simulink model "Quadrotor_Simulation"  (R2016b)
settings: Solver=VariableStepAuto  StartTime=0.0  StopTime=15  FixedStep=0.005  MaxStep=0.005  RelTol=1e-1
settings Model: Creator=Administrator  LastModifiedBy=Administrator

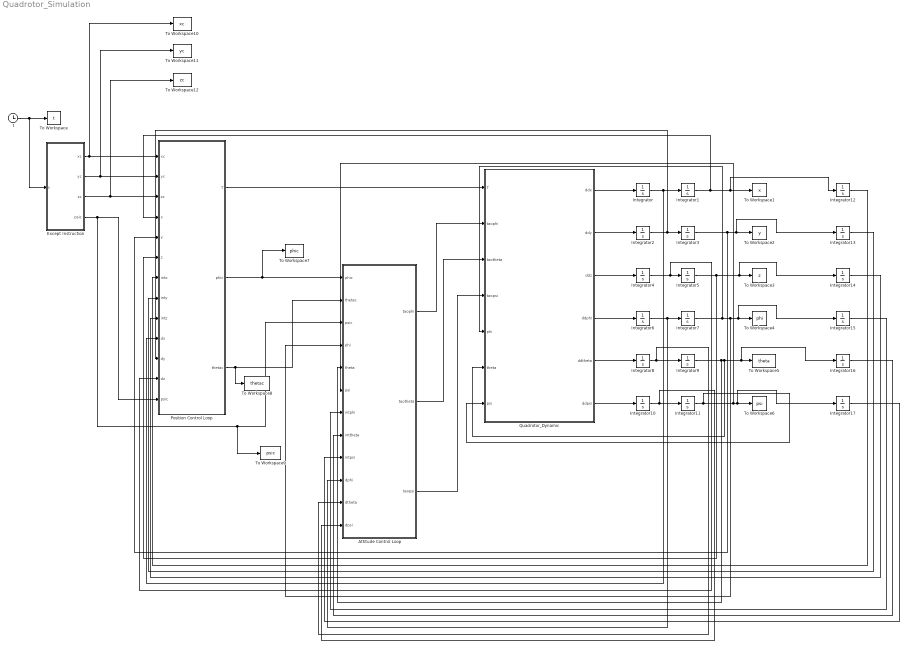
== system Quadrotor_Simulation ==
  Attitude Control Loop : Subsystem
  Except Instruction : MATLAB Function  TreatAsAtomicUnit=on
  Integrator : Integrator  InitialCondition=0.1
  Integrator{1,3,5..17} (15 alike) : Integrator
  Integrator2 : Integrator  InitialCondition=0.1
  Integrator4 : Integrator  InitialCondition=0.1
  Position Control Loop : Subsystem
  Quadrotor_Dynamic : MATLAB Function  TreatAsAtomicUnit=on
  To Workspace : ToWorkspace  VariableName=t  SampleTime=-1
  To Workspace1 : ToWorkspace  VariableName=x  SampleTime=-1
  To Workspace10 : ToWorkspace  VariableName=xc  SampleTime=-1
  To Workspace11 : ToWorkspace  VariableName=yc  SampleTime=-1
  To Workspace12 : ToWorkspace  VariableName=zc  SampleTime=-1
  To Workspace2 : ToWorkspace  VariableName=y  SampleTime=-1
  To Workspace3 : ToWorkspace  VariableName=z  SampleTime=-1
  To Workspace4 : ToWorkspace  VariableName=phi  SampleTime=-1
  To Workspace5 : ToWorkspace  VariableName=theta  SampleTime=-1
  To Workspace6 : ToWorkspace  VariableName=psi  SampleTime=-1
  To Workspace7 : ToWorkspace  VariableName=phic  SampleTime=-1
  To Workspace8 : ToWorkspace  VariableName=thetac  SampleTime=-1
  To Workspace9 : ToWorkspace  VariableName=psic  SampleTime=-1
  t : Clock
  wires:
  t/1 -> Except Instruction/1(t), To Workspace/1
  Except Instruction/1(xc) -> To Workspace10/1, Position Control Loop/1(xc)
  Except Instruction/2(yc) -> To Workspace11/1, Position Control Loop/2(yc)
  Except Instruction/3(zc) -> To Workspace12/1, Position Control Loop/3(zc)
  Except Instruction/4(psic) -> Attitude Control Loop/3(psic), To Workspace9/1, Position Control Loop/13(psic)
  Position Control Loop/2(phic) -> To Workspace7/1, Attitude Control Loop/1(phic)
  Position Control Loop/3(thetac) -> To Workspace8/1, Attitude Control Loop/2(thetac)
  Quadrotor_Dynamic/1(ddx) -> Integrator/1
  Integrator/1 -> Position Control Loop/10(dx), Integrator1/1
  Quadrotor_Dynamic/2(ddy) -> Integrator2/1
  Integrator2/1 -> Integrator3/1, Position Control Loop/11(dy)
  Quadrotor_Dynamic/3(ddz) -> Integrator4/1
  Integrator4/1 -> Position Control Loop/12(dz), Integrator5/1
  Quadrotor_Dynamic/4(ddphi) -> Integrator6/1
  Integrator6/1 -> Attitude Control Loop/10(dphi), Integrator7/1
  Quadrotor_Dynamic/5(ddtheta) -> Integrator8/1
  Integrator8/1 -> Attitude Control Loop/11(dtheta), Integrator9/1
  Quadrotor_Dynamic/6(ddpsi) -> Integrator10/1
  Integrator10/1 -> Attitude Control Loop/12(dpsi), Integrator11/1
  Integrator9/1 -> Attitude Control Loop/5(theta), Quadrotor_Dynamic/6(theta), Integrator16/1, To Workspace5/1
  Integrator11/1 -> Quadrotor_Dynamic/7(psi), Integrator17/1, To Workspace6/1, Attitude Control Loop/6(psi)
  Integrator7/1 -> Quadrotor_Dynamic/5(phi), Attitude Control Loop/4(phi), Integrator15/1, To Workspace4/1
  Integrator5/1 -> Position Control Loop/6(z), Integrator14/1, To Workspace3/1
  Integrator3/1 -> Position Control Loop/5(y), Integrator13/1, To Workspace2/1
  Integrator1/1 -> Position Control Loop/4(x), Integrator12/1, To Workspace1/1
  Position Control Loop/1(T) -> Quadrotor_Dynamic/1(T)
  Attitude Control Loop/1(taophi) -> Quadrotor_Dynamic/2(taophi)
  Attitude Control Loop/2(taotheta) -> Quadrotor_Dynamic/3(taotheta)
  Attitude Control Loop/3(taopsi) -> Quadrotor_Dynamic/4(taopsi)
  Integrator12/1 -> Position Control Loop/7(intx)
  Integrator13/1 -> Position Control Loop/8(inty)
  Integrator14/1 -> Position Control Loop/9(intz)
  Integrator15/1 -> Attitude Control Loop/7(intphi)
  Integrator16/1 -> Attitude Control Loop/8(inttheta)
  Integrator17/1 -> Attitude Control Loop/9(intpsi)

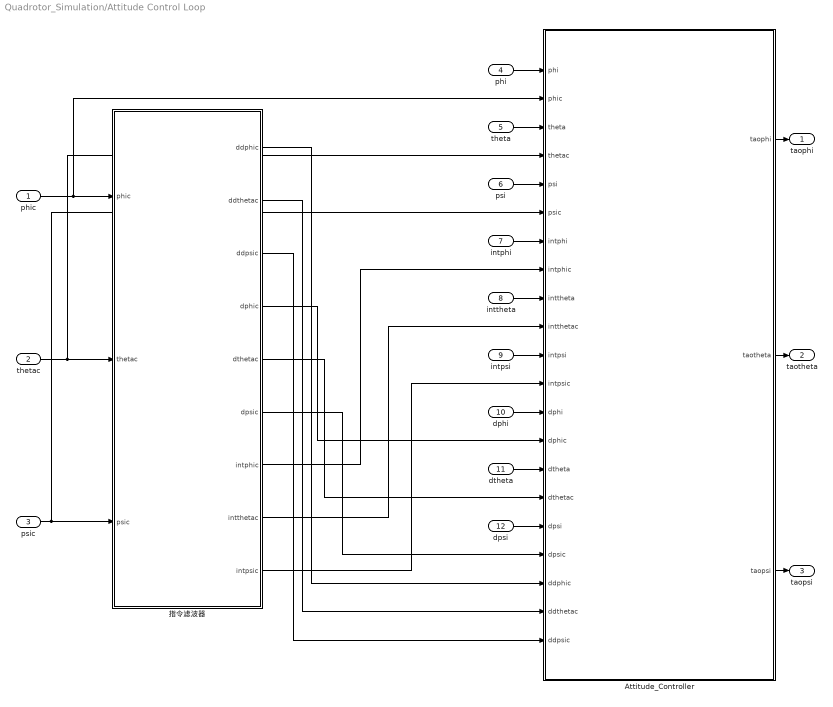
== system Quadrotor_Simulation/Attitude Control Loop ==
  phic : Inport
  thetac : Inport  Port=2
  psic : Inport  Port=3
  phi : Inport  Port=4
  theta : Inport  Port=5
  psi : Inport  Port=6
  intphi : Inport  Port=7
  inttheta : Inport  Port=8
  intpsi : Inport  Port=9
  dphi : Inport  Port=10
  dtheta : Inport  Port=11
  dpsi : Inport  Port=12
  Attitude_Controller : MATLAB Function  TreatAsAtomicUnit=on
  指令滤波器 : Subsystem
  taophi : Outport
  taotheta : Outport  Port=2
  taopsi : Outport  Port=3
  wires:
  指令滤波器/9(intpsic) -> Attitude_Controller/12(intpsic)
  指令滤波器/4(dphic) -> Attitude_Controller/14(dphic)
  dtheta/1 -> Attitude_Controller/15(dtheta)
  theta/1 -> Attitude_Controller/3(theta)
  dphi/1 -> Attitude_Controller/13(dphi)
  thetac/1 -> Attitude_Controller/4(thetac), 指令滤波器/2(thetac)
  inttheta/1 -> Attitude_Controller/9(inttheta)
  指令滤波器/7(intphic) -> Attitude_Controller/8(intphic)
  指令滤波器/5(dthetac) -> Attitude_Controller/16(dthetac)
  dpsi/1 -> Attitude_Controller/17(dpsi)
  指令滤波器/6(dpsic) -> Attitude_Controller/18(dpsic)
  指令滤波器/1(ddphic) -> Attitude_Controller/19(ddphic)
  phic/1 -> Attitude_Controller/2(phic), 指令滤波器/1(phic)
  phi/1 -> Attitude_Controller/1(phi)
  指令滤波器/8(intthetac) -> Attitude_Controller/10(intthetac)
  psi/1 -> Attitude_Controller/5(psi)
  psic/1 -> Attitude_Controller/6(psic), 指令滤波器/3(psic)
  intpsi/1 -> Attitude_Controller/11(intpsi)
  指令滤波器/3(ddpsic) -> Attitude_Controller/21(ddpsic)
  Attitude_Controller/2(taotheta) -> taotheta/1
  Attitude_Controller/3(taopsi) -> taopsi/1
  指令滤波器/2(ddthetac) -> Attitude_Controller/20(ddthetac)
  Attitude_Controller/1(taophi) -> taophi/1
  intphi/1 -> Attitude_Controller/7(intphi)

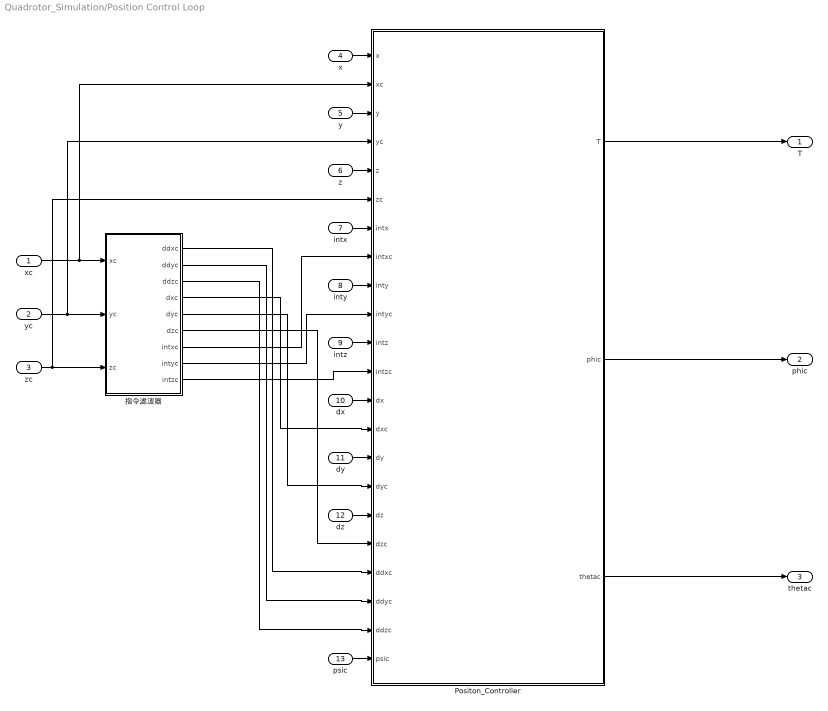
== system Quadrotor_Simulation/Position Control Loop ==
  xc : Inport
  yc : Inport  Port=2
  zc : Inport  Port=3
  x : Inport  Port=4
  y : Inport  Port=5
  z : Inport  Port=6
  intx : Inport  Port=7
  inty : Inport  Port=8
  intz : Inport  Port=9
  dx : Inport  Port=10
  dy : Inport  Port=11
  dz : Inport  Port=12
  psic : Inport  Port=13
  Positon_Controller : MATLAB Function  TreatAsAtomicUnit=on
  指令滤波器 : Subsystem
  T : Outport
  phic : Outport  Port=2
  thetac : Outport  Port=3
  wires:
  zc/1 -> Positon_Controller/6(zc), 指令滤波器/3(zc)
  yc/1 -> Positon_Controller/4(yc), 指令滤波器/2(yc)
  xc/1 -> Positon_Controller/2(xc), 指令滤波器/1(xc)
  指令滤波器/6(dzc) -> Positon_Controller/18(dzc)
  指令滤波器/8(intyc) -> Positon_Controller/10(intyc)
  指令滤波器/3(ddzc) -> Positon_Controller/21(ddzc)
  指令滤波器/7(intxc) -> Positon_Controller/8(intxc)
  指令滤波器/4(dxc) -> Positon_Controller/14(dxc)
  指令滤波器/1(ddxc) -> Positon_Controller/19(ddxc)
  指令滤波器/9(intzc) -> Positon_Controller/12(intzc)
  指令滤波器/2(ddyc) -> Positon_Controller/20(ddyc)
  指令滤波器/5(dyc) -> Positon_Controller/16(dyc)
  Positon_Controller/2(phic) -> phic/1
  Positon_Controller/3(thetac) -> thetac/1
  Positon_Controller/1(T) -> T/1
  x/1 -> Positon_Controller/1(x)
  y/1 -> Positon_Controller/3(y)
  z/1 -> Positon_Controller/5(z)
  intx/1 -> Positon_Controller/7(intx)
  inty/1 -> Positon_Controller/9(inty)
  intz/1 -> Positon_Controller/11(intz)
  dx/1 -> Positon_Controller/13(dx)
  dy/1 -> Positon_Controller/15(dy)
  dz/1 -> Positon_Controller/17(dz)
  psic/1 -> Positon_Controller/22(psic)

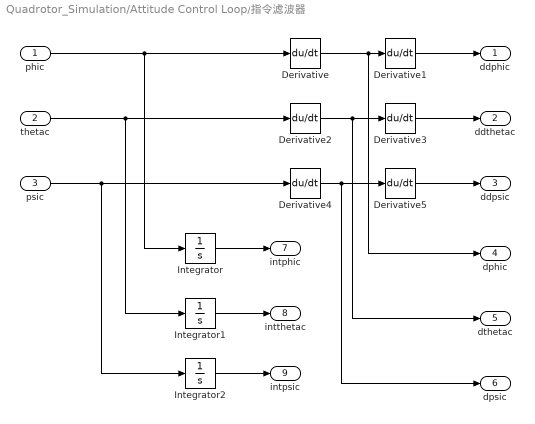
== system Quadrotor_Simulation/Attitude Control Loop/指令滤波器 ==
  phic : Inport
  thetac : Inport  Port=2
  psic : Inport  Port=3
  Derivative{,1..5} (6 alike) : Derivative
  Integrator : Integrator
  Integrator1 : Integrator
  Integrator2 : Integrator
  ddphic : Outport
  ddthetac : Outport  Port=2
  ddpsic : Outport  Port=3
  dphic : Outport  Port=4
  dthetac : Outport  Port=5
  dpsic : Outport  Port=6
  intphic : Outport  Port=7
  intthetac : Outport  Port=8
  intpsic : Outport  Port=9
  wires:
  Derivative3/1 -> ddthetac/1
  Derivative5/1 -> ddpsic/1
  Derivative1/1 -> ddphic/1
  thetac/1 -> Integrator1/1, Derivative2/1
  psic/1 -> Integrator2/1, Derivative4/1
  Derivative2/1 -> dthetac/1, Derivative3/1
  Derivative4/1 -> dpsic/1, Derivative5/1
  Derivative/1 -> dphic/1, Derivative1/1
  Integrator/1 -> intphic/1
  Integrator1/1 -> intthetac/1
  Integrator2/1 -> intpsic/1
  phic/1 -> Integrator/1, Derivative/1

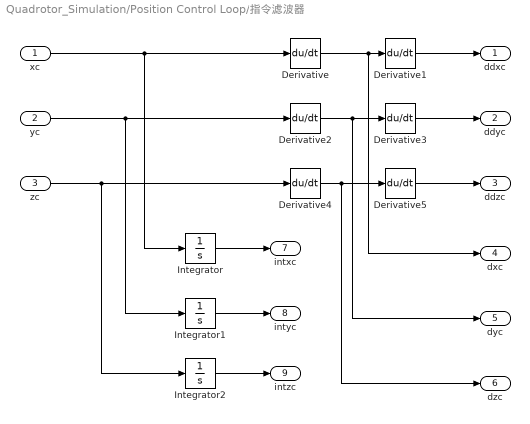
== system Quadrotor_Simulation/Position Control Loop/指令滤波器 ==
  xc : Inport
  yc : Inport  Port=2
  zc : Inport  Port=3
  Derivative{,1..5} (6 alike) : Derivative
  Integrator : Integrator
  Integrator1 : Integrator
  Integrator2 : Integrator
  ddxc : Outport
  ddyc : Outport  Port=2
  ddzc : Outport  Port=3
  dxc : Outport  Port=4
  dyc : Outport  Port=5
  dzc : Outport  Port=6
  intxc : Outport  Port=7
  intyc : Outport  Port=8
  intzc : Outport  Port=9
  wires:
  Derivative3/1 -> ddyc/1
  Derivative5/1 -> ddzc/1
  Derivative1/1 -> ddxc/1
  yc/1 -> Integrator1/1, Derivative2/1
  zc/1 -> Integrator2/1, Derivative4/1
  Derivative2/1 -> dyc/1, Derivative3/1
  Derivative4/1 -> dzc/1, Derivative5/1
  Derivative/1 -> dxc/1, Derivative1/1
  Integrator/1 -> intxc/1
  Integrator1/1 -> intyc/1
  Integrator2/1 -> intzc/1
  xc/1 -> Integrator/1, Derivative/1

== matlab function Quadrotor_Simulation/Position Control Loop/Positon_Controller ==
  data: x input; T output; xc input; y input; yc input; z input; zc input; intx input; intxc input; inty input; intyc input; intz input; intzc input; dx input; dxc input; dy input; dyc input; dz input; dzc input; ddxc input; ddyc input; ddzc input; phic output; thetac output; psic input
function [T,phic,thetac] = fcn(x,xc,y,yc,z,zc,intx,intxc,inty,intyc,intz,intzc,dx,dxc,dy,dyc,dz,dzc,ddxc,ddyc,ddzc,psic)

m = 1;
g = 9.81;

kp = 3;
ki = 0.13;
kd = 1.1;

kpx =  kp; kpy =  kp; kpz =  kp;
kix = ki; kiy = ki; kiz = ki; 
kdx = kd; kdy = kd; kdz = kd;

ex= xc - x;
ey = yc - y;
ez = zc - z;

intex = intxc - intx;
intey = intyc - inty;
intez = intzc - intz;

dex = dxc - dx;
dey = dyc - dy;
dez = dzc - dz;

%%
ddxc = 0; ddyc = 0; ddzc = 0;
%%

Ux = kpx * ex + kix * intex + kdx * dex + ddxc;
Uy = kpy * ey + kiy * intey + kdy * dey + ddyc;
Uz = kpz * ez + kiz * intez + kdz * dez + ddzc;

T = m * sqrt(Ux * Ux + Uy * Uy + (Uz + g) * (Uz + g));

temp1 = m * (Ux * sin(psic) - Uy * cos(psic)) / T;
% if temp1 > 1
%     temp1 = 1;
% elseif temp1 < -1
%     temp1 = -1;
% end
phic = asin(temp1);
% if phic > 20 * pi / 180;
%     phic = 20 * pi / 180;
% elseif phic < -20 * pi / 180
%     phic = -20 * pi / 180;
% end

temp2 = (m * Ux - T * sin(psic) * sin(phic)) / (T * cos(psic) * cos(phic));
% if temp2 > 1
%     temp2 = 1;
% elseif temp2 < -1
%     temp2 = -1;
% end
thetac = asin(temp2);
% if thetac > 20 * pi / 180
%     thetac = 20 * pi / 180;
% elseif thetac < -20 * pi / 180
%     thetac = -20 * pi / 180;
% end

== matlab function Quadrotor_Simulation/Except Instruction ==
  data: xc output; t input; yc output; zc output; psic output
function [xc,yc,zc,psic] = fcn(t)

xc = 5 * sin(t);
yc = 0.5 * sin(0.5 * t);
zc = 3;

psic = 0;

== matlab function Quadrotor_Simulation/Attitude Control Loop/Attitude_Controller ==
  data: phi input; taophi output; phic input; theta input; thetac input; psi input; psic input; intphi input; intphic input; inttheta input; intthetac input; intpsi input; intpsic input; dphi input; dphic input; dtheta input; dthetac input; dpsi input; dpsic input; ddphic input; ddthetac input; ddpsic input; taotheta output; taopsi output
function [taophi,taotheta,taopsi] = fcn(phi,phic,theta,thetac,psi,psic,intphi,intphic,inttheta,intthetac,intpsi,intpsic,dphi,dphic,dtheta,dthetac,dpsi,dpsic,ddphic,ddthetac,ddpsic)

Jx = 6.23e-3; Jy = 6.22e-3; Jz = 1.12e-3;

kp = 6;
ki = 0.6;
kd = 10;

kpphi =  kp; kptheta =  kp; kppsi =  kp;
kiphi = ki; kitheta = ki; kipsi = ki; 
kdphi = kd; kdtheta = kd; kdpsi = kd;

ephi= phic - phi;
etheta = thetac - theta;
epsi = psic - psi;

intephi = intphic - intphi;
intetheta = intthetac - inttheta;
intepsi = intpsic - intpsi;

dephi = dphic - dphi;
detheta = dthetac - dtheta;
depsi = dpsic - dpsi;

%%
ddphic = 0; ddthetac = 0; ddpsic = 0;
%%

Uphi = kpphi * ephi + kiphi * intephi + kdphi * dephi + ddphic;
Utheta = kptheta * etheta + kitheta * intetheta + kdtheta * detheta + ddthetac;
Upsi = kppsi * epsi + kipsi * intepsi + kdpsi * depsi + ddpsic;

taophi = Jx * Uphi;
taotheta = Jy * Utheta;
taopsi = Jz * Upsi;

== matlab function Quadrotor_Simulation/Quadrotor_Dynamic ==
  data: T input; ddx output; taophi input; taotheta input; taopsi input; ddy output; ddz output; ddphi output; ddtheta output; ddpsi output; phi input; theta input; psi input
function [ddx,ddy,ddz,ddphi,ddtheta,ddpsi] = fcn(T,taophi,taotheta,taopsi,phi,theta,psi)

m = 1;
g = 9.81;
Jx = 6.23e-3; Jy = 6.22e-3; Jz = 1.12e-3;


ddx = T * (cos(phi) * sin(theta) * cos(psi) + sin(phi) * sin(psi)) / m;
ddy = T * (cos(phi) * sin(theta) * sin(psi) - sin(phi) * cos(psi)) / m;
ddz = T * cos(phi) * cos(theta) / m - g;

ddphi = taophi / Jx;
ddtheta = taotheta / Jy;
ddpsi = taopsi / Jz;
